simulink model "PennyFab_OpenSystemRandomArrivals_RandomProcTimes"  (R2015a)
settings: Solver=ode45  StartTime=0.0  StopTime=10000  RelTol=1e-3
PostLoadFcn:
  | set_param(gcs, 'Location', [75 0 1300 1000]);
InitFcn:
  | warning('off','all');
StopFcn:
  | warning('on', 'all');
libraries: simeventslib x3
Description:
  | % LICENSE:  3-clause "Revised" or "New" or "Modified" BSD License.
  | % Copyright (c) 2015, Georgia Institute of Technology.
  | % All rights reserved.
  | %
  | % Redistribution and use in source and binary forms, with or without
  | % modification, are permitted provided that the following conditions are met:
  | %     * Redistributions of source code must retain the above copyright
  | %       notice, this list of conditions and the following disclaimer.
  | %     * Redistributions in binary form must reproduce the above copyright
  | %       notice, this list of conditions and the following disclaimer in the
  | %       documentation and/or other materials provided with the distribution.
  | %     * Neither the name of the Georgia Institute of Technology nor the
  | %       names of its contributors may be used to endorse or promote products
  | %       derived from this software without specific prior written permission.
  | %
  | % THIS SOFTWARE IS PROVIDED BY THE COPYRIGHT HOLDERS AND CONTRIBUTORS "AS IS" AND
  | % ANY EXPRESS OR IMPLIED WARRANTIES, INCLUDING, BUT NOT LIMITED TO, THE IMPLIED
  | % WARRANTIES OF MERCHANTABILITY AND FITNESS FOR A PARTICULAR PURPOSE ARE
  | % DISCLAIMED. IN NO EVENT SHALL THE GEORGIA INSTITUTE OF TECHNOLOGY BE LIABLE FOR
  | % ANY DIRECT, INDIRECT, INCIDENTAL, SPECIAL, EXEMPLARY, OR CONSEQUENTIAL DAMAGES
  | % (INCLUDING, BUT NOT LIMITED TO, PROCUREMENT OF SUBSTITUTE GOODS OR SERVICES;
  | % LOSS OF USE, DATA, OR PROFITS; OR BUSINESS INTERRUPTION) HOWEVER CAUSED AND
  | % ON ANY THEORY OF LIABILITY, WHETHER IN CONTRACT, STRICT LIABILITY, OR TORT
  | % (INCLUDING NEGLIGENCE OR OTHERWISE) ARISING IN ANY WAY OUT OF THE USE OF THIS
  | % SOFTWARE, EVEN IF ADVISED OF THE POSSIBILITY OF SUCH DAMAGE.
settings Model: Creator=tsprock3  LastModifiedBy=gthiers3
settings OptimizationCC: ExpressionDepthLimit=2147483647  SimCompilerOptimization=on
settings DebuggingCC: UnderspecifiedInitializationDetection=Classic  MergeDetectMultiDrivingBlocksExec=none  SolverPrmCheckMsg=warning  FcnCallInpInsideContextMsg=EnableAllAsWarning  StateNameClashWarn=warning

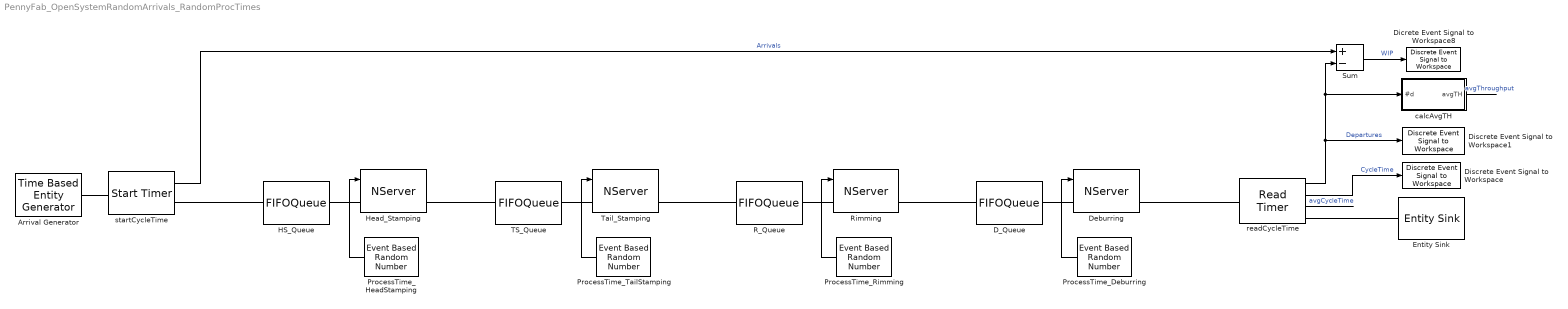
== system PennyFab_OpenSystemRandomArrivals_RandomProcTimes ==
  Arrival Generator : TimeBasedEntityGenerator  Distribution=Exponential  InitialSeed=6669  Mean=1/0.39
  D_Queue : FIFOQueue  Capacity=Inf
  Deburring : NServer  NumberOfServers=2  ServiceTimeFrom=Signal port t  ServiceTime=2  StatNumberDeparted=on
  Dicrete Event Signal to Workspace8 : simeventslib/SimEvents Sinks/Discrete Event Signal to Workspace  VariableName=WIP  SaveFormat=Structure With Time  isMonitorOnly=off  isRecordIC=off
  Discrete Event Signal to Workspace : simeventslib/SimEvents Sinks/Discrete Event Signal to Workspace  VariableName=CycleTime  SaveFormat=Structure With Time  isMonitorOnly=off  isRecordIC=off
  Discrete Event Signal to Workspace1 : simeventslib/SimEvents Sinks/Discrete Event Signal to Workspace  VariableName=Departures  SaveFormat=Structure With Time  isMonitorOnly=off  isRecordIC=off
  Entity Sink : EntitySink
  HS_Queue : FIFOQueue  Capacity=Inf
  Head_Stamping : NServer  NumberOfServers=1  ServiceTimeFrom=Signal port t  StatNumberDeparted=on
  ProcessTime_Deburring : EventBasedRandomNumber  meanExp=3  meanNorm=3  stdNorm=0.3  Seed=59337
  ProcessTime_HeadStamping : EventBasedRandomNumber  meanExp=2  meanNorm=2  stdNorm=0.2  Seed=62554
  ProcessTime_Rimming : EventBasedRandomNumber  meanExp=10  meanNorm=10  stdNorm=0.1  Seed=235
  ProcessTime_TailStamping : EventBasedRandomNumber  meanExp=5  meanNorm=5  stdNorm=0.5  Seed=3452
  R_Queue : FIFOQueue  Capacity=Inf
  Rimming : NServer  NumberOfServers=6  ServiceTimeFrom=Signal port t  ServiceTime=6  StatNumberDeparted=on
  Sum : Sum  Inputs=+-
  TS_Queue : FIFOQueue  Capacity=Inf
  Tail_Stamping : NServer  NumberOfServers=2  ServiceTimeFrom=Signal port t  ServiceTime=2  StatNumberDeparted=on
  calcAvgTH : Subsystem
  readCycleTime : ReadTimer  TimerTag=CycleTime  StatNumberDeparted=on  StatTimeElapsed=on  StatAverageTimeElapsed=on
      settings: OutputPortMap=o0,o2,o3
  startCycleTime : StartTimer  TimerTag=CycleTime  TimerStartedOption=Restart  StatNumberDeparted=on
  wires:
  readCycleTime/2 -> Discrete Event Signal to Workspace/1  "CycleTime"
  ProcessTime_HeadStamping/1 -> Head_Stamping/1
  ProcessTime_TailStamping/1 -> Tail_Stamping/1
  ProcessTime_Rimming/1 -> Rimming/1
  ProcessTime_Deburring/1 -> Deburring/1
  Sum/1 -> Dicrete Event Signal to Workspace8/1  "WIP"
  startCycleTime/1 -> Sum/1  "Arrivals"
  readCycleTime/1 -> calcAvgTH/1(#d), Sum/2, Discrete Event Signal to Workspace1/1  "Departures"
  readCycleTime/3 -> ?  "avgCycleTime"
  calcAvgTH/1(avgTH) -> ?  "avgThroughput"
  connections:
  Deburring/RConn1 -- readCycleTime/LConn1
  readCycleTime/RConn1 -- Entity Sink/LConn1
  Head_Stamping/RConn1 -- TS_Queue/LConn1
  TS_Queue/RConn1 -- Tail_Stamping/LConn1
  Tail_Stamping/RConn1 -- R_Queue/LConn1
  R_Queue/RConn1 -- Rimming/LConn1
  Rimming/RConn1 -- D_Queue/LConn1
  D_Queue/RConn1 -- Deburring/LConn1
  HS_Queue/RConn1 -- Head_Stamping/LConn1
  startCycleTime/RConn1 -- HS_Queue/LConn1
  Arrival Generator/RConn1 -- startCycleTime/LConn1

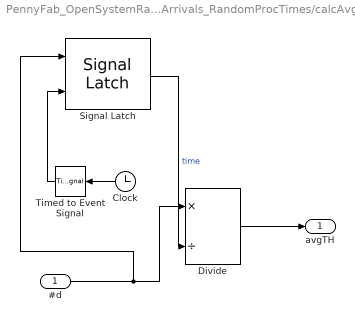
== system PennyFab_OpenSystemRandomArrivals_RandomProcTimes/calcAvgTH ==
  #d : Inport
  Clock : Clock
  Divide : Product  Inputs=*/
  Signal Latch : SignalLatch  ReadMemoryUpon=Write to memory event
      settings: InputPortMap=u0,u2  OutputPortMap=o2
  Timed to Event Signal : TimedToEventSignal
  avgTH : Outport
  wires:
  #d/1 -> Signal Latch/1, Divide/1
  Timed to Event Signal/1 -> Signal Latch/2
  Signal Latch/1 -> Divide/2  "time"
  Clock/1 -> Timed to Event Signal/1
  Divide/1 -> avgTH/1
